simulink model "m3s"  (R2022a)
settings: Solver=VariableStepAuto  StartTime=0.0  StopTime=20.0  RelTol=1e-3
values from neighbouring files (symbols this model uses):
  delta_da = 0.2    [m1.m]    (also in m2.m = 0; m3.m = 0)
  delta_dt = 0    [m1.m]    (also in m2.m; m3.m)
  delta_dy = 0    [m1.m]    (also in m2.m; m3.m)
  delta_r = 0.25    [m3.m]
  rho = 0    [m1.m]    (also in m2.m = 1; m3.m = 1)
libraries: cstblocks x2, simulink x1
settings Model: Creator=apple  LastModifiedBy=apple

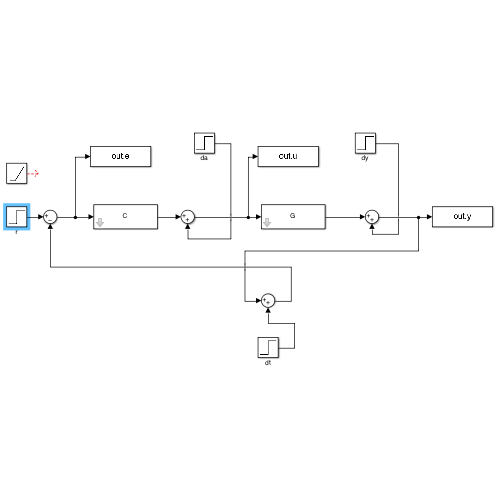
[thumbnail: Simulink's stored preview of the top-level diagram]
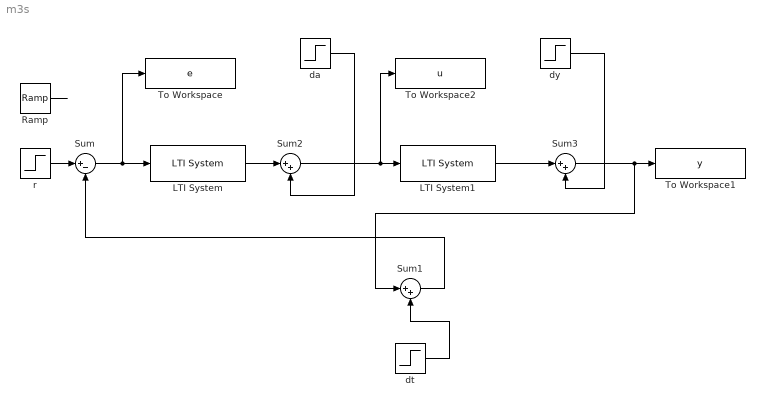
== system m3s ==
  LTI System : cstblocks/LTI System  sys=C  IC=[]
  LTI System1 : cstblocks/LTI System  sys=G  IC=[]
  Ramp : simulink/Sources/Ramp  slope=delta_r  start=0  InitialOutput=0
  Sum : Sum  Inputs=|+-
  Sum1 : Sum  Inputs=|++
  Sum2 : Sum  Inputs=|++
  Sum3 : Sum  Inputs=|++
  To Workspace : ToWorkspace  VariableName=e  SaveFormat=Timeseries  SampleTime=-1
  To Workspace1 : ToWorkspace  VariableName=y  SaveFormat=Timeseries  SampleTime=-1
  To Workspace2 : ToWorkspace  VariableName=u  SaveFormat=Timeseries  SampleTime=-1
  da : Step  Time=0  After=delta_da  SampleTime=0
  dt : Step  Time=0  After=delta_dt  SampleTime=0
  dy : Step  Time=0  After=delta_dy  SampleTime=0
  r : Step  Time=0  After=rho  SampleTime=0
  wires:
  dt/1 -> Sum1/2
  Sum/1 -> To Workspace/1, LTI System/1
  LTI System/1 -> Sum2/1
  Sum2/1 -> To Workspace2/1, LTI System1/1
  da/1 -> Sum2/2
  Sum3/1 -> Sum1/1, To Workspace1/1
  dy/1 -> Sum3/2
  LTI System1/1 -> Sum3/1
  Sum1/1 -> Sum/2
  Ramp/1 -> ?
  r/1 -> Sum/1
